simulink model "SerialParser"  (R2025b)
settings: Solver=FixedStepDiscrete  StartTime=0.0  StopTime=inf  FixedStep=0.01  RelTol=1e-3  EnableMultiTasking=on
settings Model: Creator=USER  LastModifiedBy=USER
settings SolverCC: PositivePriorityOrder=on
settings OptimizationCC: EnhancedBackFolding=on  PassReuseOutputArgsAs=Individual arguments  ZeroExternalMemoryAtStartup=off  ZeroInternalMemoryAtStartup=off  MaxStackSize=200000  OptimizeBlockOrder=speed  DifferentSizesBufferReuse=on  OptimizationCustomize=off  EfficientTunableParamExpr=on
settings DebuggingCC: ParameterTunabilityLossMsg=error
settings HardwareCC: ProdBitPerPointer=32.0  ProdBitPerSizeT=32.0  ProdBitPerPtrDiffT=32.0  ProdLargestAtomicInteger=Long  ProdLargestAtomicFloat=Double  ProdWordSize=32.0  ProdLongLongMode=on  ProdHWDeviceType=ARM Compatible->ARM Cortex-A (32-bit)  UseEmbeddedCoderFeatures=off
settings RTWCC: SystemTargetFile=ert.tlc  HardwareBoard=Raspberry Pi  TLCOptions="-aInlineSetEventsForThisBaseRateFcn=TLC_FALSE -aSuppressMultiTaskScheduler=TLC_FALSE  -aRateBasedStepFcn=0"  TemplateMakefile=ert_default_tmf  RTWVerbose=off  Toolchain=GNU GCC Embedded Linux  BuildConfiguration=Faster Runs  Description=Embedded Coder
settings CodeAppCC: ForceParamTrailComments=on  IgnoreCustomStorageClasses=off  OperatorAnnotations=on  SimulinkDataObjDesc=on  SFDataObjDesc=on  InsertBlockDesc=on
settings ERTTargetCC: ExtModeTransport=2.0  ExtModeStaticAlloc=on  ExtModeMexFile=ext_xcp  ExtModeIntrfLevel=Level2 - Open  InlinedParameterPlacement=Hierarchical  SupportNonInlinedSFcns=on  SupportVariableSizeSignals=on

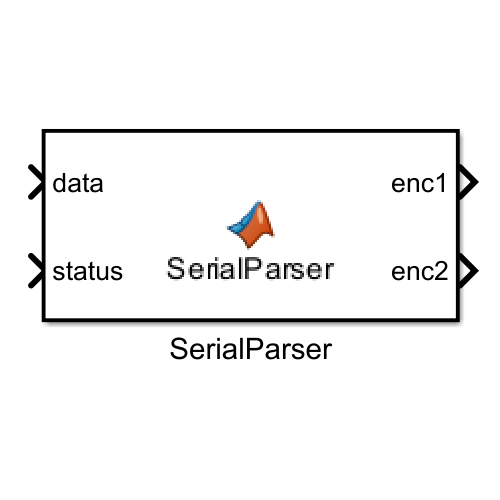
[thumbnail: Simulink's stored preview of the top-level diagram]
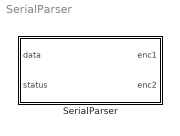
== system SerialParser ==
  SerialParser : MATLAB Function  TreatAsAtomicUnit=on

== matlab function SerialParser/SerialParser ==
  data: data input uint8 size=[10,1]; enc1 output int32 size=1; enc2 output int32 size=1; status input uint8 size=1
function [enc1, enc2] = SerialParser(data, status)

HEADER  = uint8(170);
TAIL    = uint8(85);
BUF_LEN = int32(64);

enc1 = int32(0);
enc2 = int32(0);

persistent buf len last_enc1 last_enc2
if isempty(buf)
    buf       = zeros(1, BUF_LEN, 'uint8');
    len       = int32(0);
    last_enc1 = int32(0);
    last_enc2 = int32(0);
end

enc1 = last_enc1;
enc2 = last_enc2;

if status ~= 0
    return;
end

N = numel(data);
for k = 1:N
    b = data(k);
    if len < BUF_LEN
        len = len + 1;
        buf(len) = b;
    else
        buf(1:BUF_LEN-1) = buf(2:BUF_LEN);
        buf(BUF_LEN) = b;
        len = BUF_LEN;
    end
end

i = int32(1);

while i <= len - 9
    if (buf(i) == HEADER) && (buf(i+9) == TAIL)

        b0 = uint32(buf(i+1)) ...
           + bitshift(uint32(buf(i+2)), 8) ...
           + bitshift(uint32(buf(i+3)), 16) ...
           + bitshift(uint32(buf(i+4)), 24);
        v0 = typecast(b0, 'int32');
        enc1_tmp = v0(1);

        b1 = uint32(buf(i+5)) ...
           + bitshift(uint32(buf(i+6)), 8) ...
           + bitshift(uint32(buf(i+7)), 16) ...
           + bitshift(uint32(buf(i+8)), 24);
        v1 = typecast(b1, 'int32');
        enc2_tmp = v1(1);

        last_enc1 = enc1_tmp;
        last_enc2 = enc2_tmp;
        enc1 = last_enc1;
        enc2 = last_enc2;

        leftover = len - (i + 9);
        if leftover > 0
            buf(1:leftover) = buf((i+10):(i+9+leftover));
        end
        len = leftover;

        i = int32(1);
    else
        i = i + 1;
    end
end
